simulink model "Coupled_GP_fit"  (R2018b)
settings: Solver=FixedStepAuto  StartTime=0.0  StopTime=t_end  FixedStep=ts  MinStep=1/1e5  RelTol=1e-3
values from neighbouring files (symbols this model uses):
  a0 = omega_n^3    (= 248050213.442)    [TwoLink_init.m]    (also in init.m = 31006276.6803)
  a1 = 3*omega_n^2    (= 1184352.52813)    [TwoLink_init.m]    (also in init.m = 296088.132033)
  a2 = 3*omega_n    (= 1884.95559215)    [TwoLink_init.m]    (also in init.m = 942.477796077)
  b1 = b(:,1)    [init.m]
  b2 = b(:,2)    [init.m]
  D = 50    [Train_SSGP.m]    (also in init.m = 21)
  g = 9.81    [init.m]
  h = 1    [init.m]
  I_limit = 2000    [TwoLink_init.m]
  L1 = 1    [init.m]
  L2 = 1    [init.m]
  m1 = 1    [init.m]
  m2 = 5    [init.m]
  mu_X = mean(xTrain')    [Train_SSGP.m]    (also in init.m = zeros(1,size(n,2)))
  mu_Y = mean(yTrain')    [Train_SSGP.m]    (also in init.m = zeros(1,size(Q,2)))
  N = size(xTrain,2)    [Train_SSGP.m]    (also in init.m = length(noiseSignal))
  r = 5e3    (= 5000)    [init.m]
  R1 = squeeze(R(1,:,:))    [init.m]
  R2 = squeeze(R(2,:,:))    [init.m]
  s = xTrain(:,i_s)'    [Train_SSGP.m]    (also in TwoLink_init.m = tf('s'))
  seed = randi(1e6)    [init.m]
  sf1 = sf(1)    [init.m]
  sf2 = sf(2)    [init.m]
  sig_X = std(xTrain')    [Train_SSGP.m]    (also in init.m = ones(1,size(n,2)))
  sig_Y = std(yTrain')    [Train_SSGP.m]    (also in init.m = ones(1,size(n,2)))
  SIGMA1 = squeeze(SIGMA(1,:,:))    [init.m]
  SIGMA2 = squeeze(SIGMA(2,:,:))    [init.m]
  sp_ts = 2.5    [init.m]
  t_learn = 0    [init.m]
  t_predict = 50    [init.m]
  tm = 2    [init.m]
  ts = 1/1000    (= 0.001)    [Train_SSGP.m]    (also in TwoLink_init.m; init.m)
  w1 = w(:,1)    [init.m]
  w2 = w(:,2)    [init.m]
  X = squeeze(xTraining(:,1,:))'    [init.m]    (also in plot_train_data.m = squeeze(input_vector.Data(:,:,ts_index)))
  Y = yTraining    [init.m]
undefined symbols (not defined in the file or in its folder): DiscIntNeverNeededParam, FF, noise, PID, Z
libraries: sm_lib x13, simulink x6, nesl_utility x5
(part 1 of 2)
settings Model: Creator=wout7  LastModifiedBy=wout7
settings DataIOCC: SaveFormat=StructureWithTime
settings OptimizationCC: BlockReduction=off  EfficientMapNaN2IntZero=off  SimCompilerOptimization=on
settings HardwareCC: TargetBitPerPointer=64  TargetBitPerSizeT=64  TargetBitPerPtrDiffT=64  TargetLongLongMode=on  TargetIntDivRoundTo=Zero  TargetEndianess=LittleEndian  TargetWordSize=64  TargetHWDeviceType=MATLAB Host  ProdEqTarget=off
settings SFSimCC: SimCustomSourceCode=solve_chol.c  MATLABDynamicMemAllocThreshold=98304
settings CodeAppCC: MaxIdLength=128
settings GRTTargetCC: TargetLangStandard=C89/C90 (ANSI)  CombineOutputUpdateFcns=off  GRTInterface=on

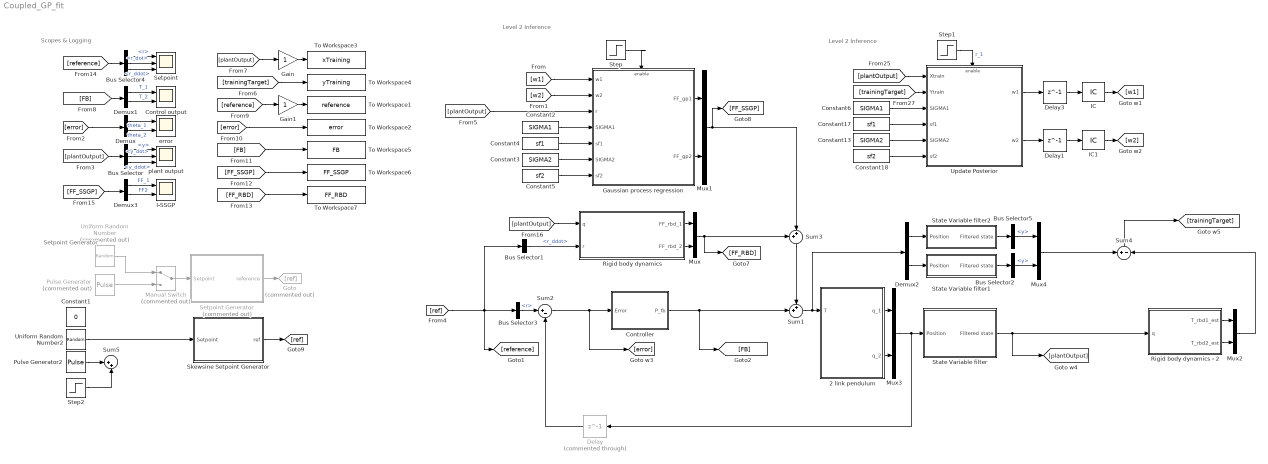
== system Coupled_GP_fit ==
  note: Level 2 Inference
  note: Scopes & Logging
  note: Level 2 Inference
  note: Setpoint Generator
  2 link pendulum : Subsystem
  Bus Selector : BusSelector  OutputSignals=y,y_dot,y_ddot
  Bus Selector1 : BusSelector  OutputSignals=r_ddot
  Bus Selector2 : BusSelector  OutputSignals=y
  Bus Selector3 : BusSelector  OutputSignals=r
  Bus Selector4 : BusSelector  OutputSignals=r,r_dot,r_ddot
  Bus Selector5 : BusSelector  OutputSignals=y
  Constant1 : Constant  Value=0  SampleTime=sp_ts
  Constant13 : Constant  Value=SIGMA2
  Constant17 : Constant  Value=sf1
  Constant18 : Constant  Value=sf2
  Constant2 : Constant  Value=SIGMA1
  Constant3 : Constant  Value=SIGMA2
  Constant4 : Constant  Value=sf1
  Constant5 : Constant  Value=sf2
  Constant6 : Constant  Value=SIGMA1
  Control output : Scope  NumInputPorts=2
  Controller : Subsystem
  Delay : Delay  Commented=through  DelayLength=1  InitialCondition=0
  Delay1 : Delay  DelayLength=1  InitialCondition=0
  Delay3 : Delay  DelayLength=1  InitialCondition=0
  Demux{,1..3} (4 alike) : Demux  Outputs=2
  Gain : Gain
  Gain1 : Gain
  Gaussian process regression : Subsystem
  Goto : Goto  Commented=on  GotoTag=ref
  I-SSGP : Scope  NumInputPorts=2
  IC : InitialCondition  Value=w1
  IC1 : InitialCondition  Value=w2
  Manual Switch : ManualSwitch  Commented=on
  Mux{,1..4} (5 alike) : Mux  Inputs=2
  Pulse Generator : DiscretePulseGenerator  Commented=on  PulseType=Time based  Amplitude=20*pi/180  Period=sp_ts  PulseWidth=50
  Pulse Generator2 : DiscretePulseGenerator  Amplitude=80*pi/180  Period=4  PulseWidth=2  SampleTime=sp_ts
  Rigid body dynamics : Subsystem
  Rigid body dynamics - 2 : Subsystem
  Setpoint : Scope  NumInputPorts=3
  Setpoint Generator : Subsystem  Commented=on
  Skewsine Setpoint Generator : Subsystem
  State Variable filter : Subsystem
  State Variable filter1 : Subsystem
  State Variable filter2 : Subsystem
  Step : Step  Time=t_predict  SampleTime=ts
  Step1 : Step  Time=t_learn  SampleTime=ts
  Step2 : Step  Time=sp_ts  After=-40*pi/180  SampleTime=sp_ts
  Sum1 : Sum  Inputs=++|
  Sum2 : Sum  Inputs=|+-
  Sum3 : Sum  Inputs=++|
  Sum4 : Sum  Inputs=+|-
  Sum5 : Sum  Inputs=|++
  To Workspace1 : ToWorkspace  VariableName=reference  SampleTime=-1
  To Workspace2 : ToWorkspace  VariableName=error  SampleTime=-1
  To Workspace3 : ToWorkspace  VariableName=xTraining  SampleTime=-1
  To Workspace4 : ToWorkspace  VariableName=yTraining  SampleTime=-1
  To Workspace5 : ToWorkspace  VariableName=FB  SampleTime=-1
  To Workspace6 : ToWorkspace  VariableName=FF_SSGP  SampleTime=-1
  To Workspace7 : ToWorkspace  VariableName=FF_RBD  SampleTime=-1
  Uniform Random Number : UniformRandomNumber  Commented=on  Minimum=-50*pi/180  Maximum=50*pi/180  Seed=seed  SampleTime=sp_ts
  Uniform Random Number2 : UniformRandomNumber  Minimum=-50*pi/180  Maximum=50*pi/180  Seed=seed  SampleTime=sp_ts
  Update Posterior : Subsystem
  error : Scope  NumInputPorts=2
  plant output : Scope  NumInputPorts=3
  wires:
  2 link pendulum/1(q_1) -> Mux3/1
  2 link pendulum/2(q_2) -> Mux3/2
  Sum1/1 -> Demux2/1, 2 link pendulum/1(T)
  Rigid body dynamics/1(FF_rbd_1) -> Mux/1
  Rigid body dynamics/2(FF_rbd_2) -> Mux/2
  Rigid body dynamics - 2/1(T_rbd1_est) -> Mux2/1
  Rigid body dynamics - 2/2(T_rbd2_est) -> Mux2/2
  Mux1/1 -> Sum3/2, [FF_SSGP]
  Sum4/1 -> [trainingTarget]
  Gaussian process regression/2(FF_gp2) -> Mux1/2
  Gaussian process regression/1(FF_gp1) -> Mux1/1
  Step/1 -> Gaussian process regression/Enable
  [w1] -> Gaussian process regression/1(w1)
  Update Posterior/1(w1) -> Delay3/1
  IC/1 -> [w1]
  IC1/1 -> [w2]
  [w2] -> Gaussian process regression/2(w2)
  Update Posterior/2(w2) -> Delay1/1
  Delay3/1 -> IC/1
  Delay1/1 -> IC1/1
  Mux2/1 -> Sum4/2
  Pulse Generator/1 -> Manual Switch/2
  Uniform Random Number/1 -> Manual Switch/1
  Controller/1(P_fb) -> Sum1/2, [FB]
  Mux/1 -> Sum3/1, [FF_RBD]
  [ref] -> Bus Selector1/1, [reference], Bus Selector3/1
  Sum3/1 -> Sum1/1
  Mux3/1 -> Delay/1, State Variable filter/1(Position)
  Bus Selector3/1 -> Sum2/1  "<r>"
  Bus Selector1/1 -> Rigid body dynamics/2(r)  "<r_ddot>"
  Setpoint Generator/1(reference) -> Goto/1
  Manual Switch/1 -> Setpoint Generator/1(Setpoint)
  Sum2/1 -> Controller/1(Error), [error]
  Delay/1 -> Sum2/2
  Step1/1 -> Update Posterior/Enable  "r_1"
  [plantOutput] -> Bus Selector/1
  Bus Selector/1 -> plant output/1  "<y>"
  Bus Selector/2 -> plant output/2  "<y_dot>"
  Bus Selector/3 -> plant output/3  "<y_ddot>"
  [error] -> Demux/1
  Demux/1 -> error/1  "theta_1"
  Demux/2 -> error/2  "theta_2"
  [trainingTarget] -> To Workspace4/1
  [plantOutput] -> Gain/1
  [reference] -> Gain1/1
  Demux1/1 -> Control output/1  "T_1"
  Demux1/2 -> Control output/2  "T_2"
  [FB] -> Demux1/1
  Gain/1 -> To Workspace3/1
  Gain1/1 -> To Workspace1/1
  [error] -> To Workspace2/1
  [FB] -> To Workspace5/1
  [FF_SSGP] -> To Workspace6/1
  [FF_RBD] -> To Workspace7/1
  [reference] -> Bus Selector4/1
  Bus Selector4/1 -> Setpoint/1  "<r>"
  Bus Selector4/2 -> Setpoint/2  "<r_dot>"
  Bus Selector4/3 -> Setpoint/3  "<r_ddot>"
  Skewsine Setpoint Generator/1(ref) -> [ref]
  Pulse Generator2/1 -> Sum5/1
  Step2/1 -> Sum5/2
  Uniform Random Number2/1 -> Skewsine Setpoint Generator/1(Setpoint)
  State Variable filter/1(Filtered state) -> Rigid body dynamics - 2/1(q), [plantOutput]
  Demux3/2 -> I-SSGP/2  "FF2"
  Demux3/1 -> I-SSGP/1  "FF_1"
  [FF_SSGP] -> Demux3/1
  Constant2/1 -> Gaussian process regression/4(SIGMA1)
  Constant4/1 -> Gaussian process regression/5(sf1)
  Constant6/1 -> Update Posterior/3(SIGMA1)
  Constant17/1 -> Update Posterior/4(sf1)
  Constant13/1 -> Update Posterior/5(SIGMA2)
  Constant18/1 -> Update Posterior/6(sf2)
  Constant3/1 -> Gaussian process regression/6(SIGMA2)
  Constant5/1 -> Gaussian process regression/7(sf2)
  [plantOutput] -> Update Posterior/1(Xtrain)
  [trainingTarget] -> Update Posterior/2(Ytrain)
  [plantOutput] -> Rigid body dynamics/1(q)
  State Variable filter1/1(Filtered state) -> Bus Selector2/1
  Mux4/1 -> Sum4/1
  Demux2/1 -> State Variable filter2/1(Position)
  Demux2/2 -> State Variable filter1/1(Position)
  Bus Selector5/1 -> Mux4/1  "<y>"
  State Variable filter2/1(Filtered state) -> Bus Selector5/1
  Bus Selector2/1 -> Mux4/2  "<y>"
  [plantOutput] -> Gaussian process regression/3(r)

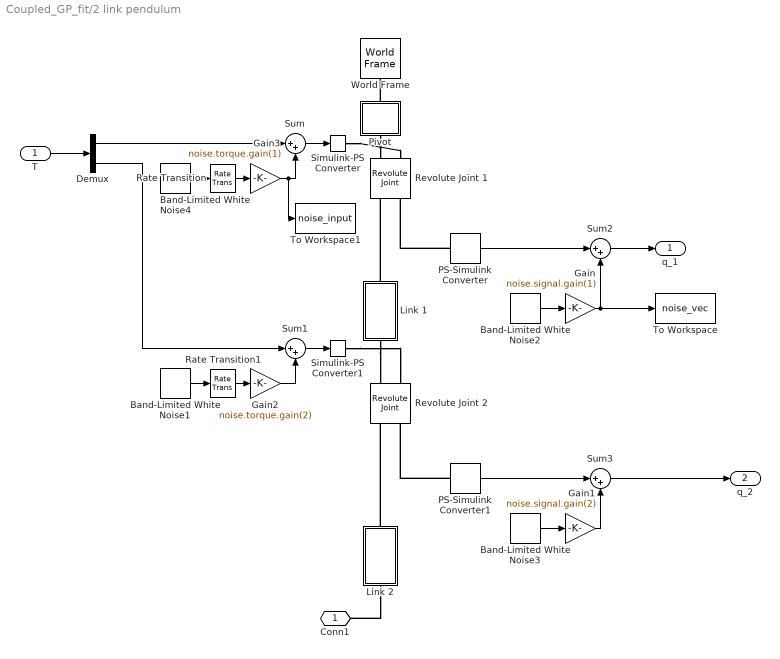
== system Coupled_GP_fit/2 link pendulum ==
  T : Inport
  Band-Limited White Noise1 : simulink/Sources/Band-Limited White Noise  Cov=noise.torque.power(2)  Ts=noise.sampleTime(1)  seed=[23341]
  Band-Limited White Noise2 : simulink/Sources/Band-Limited White Noise  Cov=noise.signal.power(1)  Ts=noise.sampleTime(2)  seed=[23341]
  Band-Limited White Noise3 : simulink/Sources/Band-Limited White Noise  Cov=noise.signal.power(2)  Ts=noise.sampleTime(2)  seed=[23341]
  Band-Limited White Noise4 : simulink/Sources/Band-Limited White Noise  Cov=noise.torque.power(1)  Ts=noise.sampleTime(1)  seed=[23341]
  Demux : Demux  Outputs=2
  Gain : Gain  Gain=noise.signal.gain(1)
  Gain1 : Gain  Gain=noise.signal.gain(2)
  Gain2 : Gain  Gain=noise.torque.gain(2)
  Gain3 : Gain  Gain=noise.torque.gain(1)
  Link 1 : Subsystem  Tag=CustomStyle
  Link 2 : Subsystem  Tag=CustomStyle
  PS-Simulink Converter : nesl_utility/PS-Simulink Converter  PhysicalDomain=network_engine_domain  SubClassName=ps_output  LeftPortType=input  RightPortType=output  PseudoPeriodic=off  Frequencies=[]  Unit=rad  AffineConversion=off
  PS-Simulink Converter1 : nesl_utility/PS-Simulink Converter  PhysicalDomain=network_engine_domain  SubClassName=ps_output  LeftPortType=input  RightPortType=output  PseudoPeriodic=off  Frequencies=[]  Unit=rad  AffineConversion=off
  Pivot : Subsystem  Tag=CustomStyle
  Rate Transition : RateTransition  OutPortSampleTime=ts
  Rate Transition1 : RateTransition  OutPortSampleTime=ts
  Revolute Joint 1 : sm_lib/Joints/Revolute Joint  SenseConstraintForce=off  SenseConstraintForceX=off  SenseConstraintForceY=off  SenseConstraintForceZ=off  SenseConstraintTorque=off  SenseConstraintTorqueX=off  SenseConstraintTorqueY=off  SenseConstraintTorqueZ=off  SenseTotalForce=off  SenseTotalForceX=off  SenseTotalForceY=off  SenseTotalForceZ=off  SenseTotalTorque=off  SenseTotalTorqueX=off  SenseTotalTorqueY=off  SenseTotalTorqueZ=off  CompositeWrenchDir=FollowerOnBase  CompositeWrenchFrame=BaseFrame  EquilibriumPosition=0  EquilibriumPositionUnits=rad  SpringStiffness=C_k1  SpringStiffnessUnits=N*m/rad  DampingCoefficient=C_d1  DampingCoefficientUnits=N*m/(rad/s)  TorqueActuationMode=InputTorque  MotionActuationMode=ComputedMotion  SensePosition=on  SenseVelocity=off  SenseAcceleration=off  SenseTorqueForce=off  PositionTargetSpecify=on  PositionTargetPriority=High  PositionTargetValue=theta1_0  PositionTargetValueUnits=deg  VelocityTargetSpecify=off  VelocityTargetPriority=High  VelocityTargetValue=0  VelocityTargetValueUnits=rad/s
  Revolute Joint 2 : sm_lib/Joints/Revolute Joint  SenseConstraintForce=off  SenseConstraintForceX=off  SenseConstraintForceY=off  SenseConstraintForceZ=off  SenseConstraintTorque=off  SenseConstraintTorqueX=off  SenseConstraintTorqueY=off  SenseConstraintTorqueZ=off  SenseTotalForce=off  SenseTotalForceX=off  SenseTotalForceY=off  SenseTotalForceZ=off  SenseTotalTorque=off  SenseTotalTorqueX=off  SenseTotalTorqueY=off  SenseTotalTorqueZ=off  CompositeWrenchDir=FollowerOnBase  CompositeWrenchFrame=BaseFrame  EquilibriumPosition=0  EquilibriumPositionUnits=rad  SpringStiffness=C_k1  SpringStiffnessUnits=N*m/rad  DampingCoefficient=C_d1  DampingCoefficientUnits=N*m/(rad/s)  TorqueActuationMode=InputTorque  MotionActuationMode=ComputedMotion  SensePosition=on  SenseVelocity=off  SenseAcceleration=off  SenseTorqueForce=off  PositionTargetSpecify=on  PositionTargetPriority=High  PositionTargetValue=theta2_0  PositionTargetValueUnits=deg  VelocityTargetSpecify=off  VelocityTargetPriority=High  VelocityTargetValue=0  VelocityTargetValueUnits=rad/s
  Simulink-PS Converter : nesl_utility/Simulink-PS Converter  PhysicalDomain=network_engine_domain  SubClassName=ps_input  LeftPortType=input  RightPortType=output  PseudoPeriodic=off  Frequencies=[]  NoiseDistribution=none  NoiseParameters=[]  Unit=1  AffineConversion=off  FilteringAndDerivatives=provide  SimscapeFilterOrder=1  InputFilterTimeConstant=0.001  UdotUserProvided=0
  Simulink-PS Converter1 : nesl_utility/Simulink-PS Converter  PhysicalDomain=network_engine_domain  SubClassName=ps_input  LeftPortType=input  RightPortType=output  PseudoPeriodic=off  Frequencies=[]  NoiseDistribution=none  NoiseParameters=[]  Unit=1  AffineConversion=off  FilteringAndDerivatives=provide  SimscapeFilterOrder=1  InputFilterTimeConstant=0.001  UdotUserProvided=0
  Sum{,1..3} (4 alike) : Sum  Inputs=|++
  To Workspace : ToWorkspace  VariableName=noise_vec  SaveFormat=Timeseries  SampleTime=-1
  To Workspace1 : ToWorkspace  VariableName=noise_input  SaveFormat=Timeseries  SampleTime=-1
  World Frame : sm_lib/Frames and Transforms/World Frame
  Conn1 : PMIOPort  Side=Left
  q_1 : Outport  SampleTime=ts
  q_2 : Outport  Port=2  SampleTime=ts
  wires:
  T/1 -> Demux/1
  Band-Limited White Noise1/1 -> Rate Transition1/1
  Demux/1 -> Sum/1
  Sum/1 -> Simulink-PS Converter/1
  Demux/2 -> Sum1/1
  Band-Limited White Noise2/1 -> Gain/1
  Sum2/1 -> q_1/1
  Band-Limited White Noise3/1 -> Gain1/1
  Sum3/1 -> q_2/1
  Gain/1 -> To Workspace/1, Sum2/2
  Gain1/1 -> Sum3/2
  Gain2/1 -> Sum1/2
  Gain3/1 -> Sum/2, To Workspace1/1
  Sum1/1 -> Simulink-PS Converter1/1
  Band-Limited White Noise4/1 -> Rate Transition/1
  Rate Transition/1 -> Gain3/1
  Rate Transition1/1 -> Gain2/1
  PS-Simulink Converter/1 -> Sum2/1
  PS-Simulink Converter1/1 -> Sum3/1
  connections:
  PS-Simulink Converter/LConn1 -- Revolute Joint 1/RConn2
  Link 2/RConn1 -- Revolute Joint 2/RConn1
  Pivot/LConn1 -- World Frame/RConn1
  Simulink-PS Converter/RConn1 -- Revolute Joint 1/LConn2
  Link 1/RConn1 -- Revolute Joint 1/RConn1
  Pivot/RConn1 -- Revolute Joint 1/LConn1
  PS-Simulink Converter1/LConn1 -- Revolute Joint 2/RConn2
  Link 1/LConn1 -- Revolute Joint 2/LConn1
  Link 2/LConn1 -- Conn1/RConn1
  Simulink-PS Converter1/RConn1 -- Revolute Joint 2/LConn2

== system Coupled_GP_fit/Controller ==
  Error : Inport
  Demux : Demux  Outputs=2
  Demux1 : Demux  Commented=on  Outputs=2
  Goto : Goto  Commented=on
  Mux : Mux  Inputs=2
  Mux1 : Mux  Commented=on  Inputs=2
  PID 1 : Subsystem  Commented=on
  PID 2 : Subsystem  Commented=on
  PID Controller : simulink/Continuous/PID Controller  Controller=PID  Form=Parallel  TimeDomain=Discrete-time  SampleTime=-1  IntegratorMethod=Forward Euler  FilterMethod=Forward Euler  ControllerParametersSource=internal  P=PID(1).kp*PID(1).sign*PID(1).sign  I=PID(1).ki*PID(1).sign  D=PID(1).kd*PID(1).sign  UseFilter=on  N=PID(1).N*PID(1).sign  TunerSelectOption=Transfer Function Based (PID Tuner App)  InitialConditionSource=internal  InitialConditionForIntegrator=0  InitialConditionForFilter=0  DifferentiatorICPrevScaledInput=0  ExternalReset=none  TrackingMode=off  Kt=1  LimitOutput=off  UpperSaturationLimit=inf  LowerSaturationLimit=-inf  LinearizeAsGain=on  AntiWindupMode=none  Kb=1  POutMin=[]  POutMax=[]  IOutMin=[]  IOutMax=[]  DOutMin=[]  DOutMax=[]  NOutMin=[]  NOutMax=[]  SumOutMin=[]  SumOutMax=[]  SaturationOutMin=[]  SaturationOutMax=[]  PParamMin=[]  PParamMax=[]  IParamMin=[]  IParamMax=[]  DParamMin=[]  DParamMax=[]  NParamMin=[]  NParamMax=[]  KbParamMin=[]  KbParamMax=[]  KtParamMin=[]  KtParamMax=[]  KbOutMin=[]  KbOutMax=[]  KtOutMin=[]  KtOutMax=[]  IntegratorOutMin=[]  IntegratorOutMax=[]  FilterOutMin=[]  FilterOutMax=[]  SumI1OutMin=[]  SumI1OutMax=[]  SumI2OutMin=[]  SumI2OutMax=[]  SumI3OutMin=[]  SumI3OutMax=[]  SumI4OutMin=[]  SumI4OutMax=[]  SumDOutMin=[]  SumDOutMax=[]  DifferentiatorOutMin=[]  DifferentiatorOutMax=[]  FilterDiffOutCoefMin=[]  FilterDiffOutCoefMax=[]  ReciprocalOutMin=[]  ReciprocalOutMax=[]  SumDenOutMin=[]  SumDenOutMax=[]  SumNumOutMin=[]  SumNumOutMax=[]  DivideOutMin=[]  DivideOutMax=[]  IntegratorContinuousStateAttributes=''  IntegratorStateMustResolveToSignalObject=off  IntegratorRTWStateStorageClass=Auto  FilterContinuousStateAttributes=''  FilterStateMustResolveToSignalObject=off  FilterRTWStateStorageClass=Auto  ParallelPVariant=InternalParameters  IdealPVariant=Disabled  IVariant=InternalParameters  DVariant=InternalParameters  IntegratorVariant=Discrete  SatVariant=Disabled  AWVariant=Passthrough  PCopyVariant=Disabled  TRVariant=Disabled  FdbkBlocksVariant=Forward  IdealPFdbkVariant=Disabled  SatFdbkVariant=Disabled  DerivativeFilterVariant=ForwardEulerFilter  NVariant=InternalParameters  NCopyVariant=Disabled  FilterICVariant=InternalICsFilter  IntegratorICVariant=InternalICs  ExternalResetVariant=Disabled  TRSumVariant=Passthrough  SumFdbkVariant=Disabled  SumVariant=Sum_PID
  PID Controller1 : simulink/Continuous/PID Controller  Controller=PID  Form=Parallel  TimeDomain=Discrete-time  SampleTime=-1  IntegratorMethod=Forward Euler  FilterMethod=Forward Euler  ControllerParametersSource=internal  P=PID(2).kp*PID(2).sign*PID(2).sign  I=PID(2).ki*PID(2).sign  D=PID(2).kd*PID(2).sign  UseFilter=on  N=PID(2).N*PID(2).sign  TunerSelectOption=Transfer Function Based (PID Tuner App)  InitialConditionSource=internal  InitialConditionForIntegrator=0  InitialConditionForFilter=0  DifferentiatorICPrevScaledInput=0  ExternalReset=none  TrackingMode=off  Kt=1  LimitOutput=off  UpperSaturationLimit=inf  LowerSaturationLimit=-inf  LinearizeAsGain=on  AntiWindupMode=none  Kb=1  POutMin=[]  POutMax=[]  IOutMin=[]  IOutMax=[]  DOutMin=[]  DOutMax=[]  NOutMin=[]  NOutMax=[]  SumOutMin=[]  SumOutMax=[]  SaturationOutMin=[]  SaturationOutMax=[]  PParamMin=[]  PParamMax=[]  IParamMin=[]  IParamMax=[]  DParamMin=[]  DParamMax=[]  NParamMin=[]  NParamMax=[]  KbParamMin=[]  KbParamMax=[]  KtParamMin=[]  KtParamMax=[]  KbOutMin=[]  KbOutMax=[]  KtOutMin=[]  KtOutMax=[]  IntegratorOutMin=[]  IntegratorOutMax=[]  FilterOutMin=[]  FilterOutMax=[]  SumI1OutMin=[]  SumI1OutMax=[]  SumI2OutMin=[]  SumI2OutMax=[]  SumI3OutMin=[]  SumI3OutMax=[]  SumI4OutMin=[]  SumI4OutMax=[]  SumDOutMin=[]  SumDOutMax=[]  DifferentiatorOutMin=[]  DifferentiatorOutMax=[]  FilterDiffOutCoefMin=[]  FilterDiffOutCoefMax=[]  ReciprocalOutMin=[]  ReciprocalOutMax=[]  SumDenOutMin=[]  SumDenOutMax=[]  SumNumOutMin=[]  SumNumOutMax=[]  DivideOutMin=[]  DivideOutMax=[]  IntegratorContinuousStateAttributes=''  IntegratorStateMustResolveToSignalObject=off  IntegratorRTWStateStorageClass=Auto  FilterContinuousStateAttributes=''  FilterStateMustResolveToSignalObject=off  FilterRTWStateStorageClass=Auto  ParallelPVariant=InternalParameters  IdealPVariant=Disabled  IVariant=InternalParameters  DVariant=InternalParameters  IntegratorVariant=Discrete  SatVariant=Disabled  AWVariant=Passthrough  PCopyVariant=Disabled  TRVariant=Disabled  FdbkBlocksVariant=Forward  IdealPFdbkVariant=Disabled  SatFdbkVariant=Disabled  DerivativeFilterVariant=ForwardEulerFilter  NVariant=InternalParameters  NCopyVariant=Disabled  FilterICVariant=InternalICsFilter  IntegratorICVariant=InternalICs  ExternalResetVariant=Disabled  TRSumVariant=Passthrough  SumFdbkVariant=Disabled  SumVariant=Sum_PID
  P_fb : Outport
  wires:
  Demux/2 -> PID Controller1/1
  Demux/1 -> PID Controller/1
  Error/1 -> Demux1/1, Demux/1
  PID Controller1/1 -> Mux/2  "T_fb2"
  PID Controller/1 -> Mux/1  "T_fb1"
  Demux1/1 -> PID 1/1(In1)
  Demux1/2 -> PID 2/1(In1)
  PID 1/1(Out1) -> Mux1/1
  PID 2/1(Out1) -> Mux1/2
  Mux1/1 -> Goto/1
  [A] -> P_fb/1
  Mux/1 -> [A]

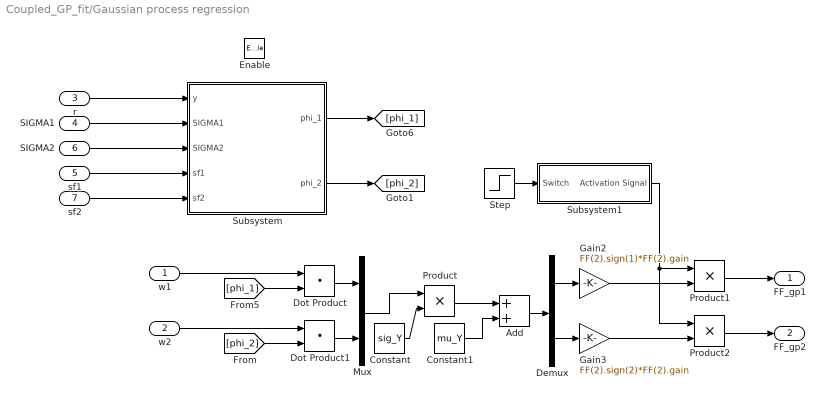
== system Coupled_GP_fit/Gaussian process regression ==
  w1 : Inport
  w2 : Inport  Port=2
  r : Inport  Port=3
  SIGMA1 : Inport  Port=4
  sf1 : Inport  Port=5
  SIGMA2 : Inport  Port=6
  sf2 : Inport  Port=7
  Enable : EnablePort
  Add : Sum
  Constant : Constant  Value=sig_Y  VectorParams1D=off  SampleTime=ts
  Constant1 : Constant  Value=mu_Y  VectorParams1D=off  SampleTime=ts
  Demux : Demux  Outputs=2
  Dot Product : DotProduct  OutDataTypeStr=Inherit: Inherit via internal rule
  Dot Product1 : DotProduct  OutDataTypeStr=Inherit: Inherit via internal rule
  Gain2 : Gain  Gain=FF(2).sign(1)*FF(2).gain
  Gain3 : Gain  Gain=FF(2).sign(2)*FF(2).gain
  Mux : Mux  Inputs=2
  Product : Product
  Product1 : Product
  Product2 : Product
  Step : Step  Time=t_predict  SampleTime=ts
  Subsystem : Subsystem
  Subsystem1 : Subsystem
  FF_gp1 : Outport  SampleTime=ts
  FF_gp2 : Outport  Port=2  SampleTime=ts
  wires:
  w1/1 -> Dot Product/1
  w2/1 -> Dot Product1/1
  [phi_2] -> Dot Product1/2
  [phi_1] -> Dot Product/2
  SIGMA2/1 -> Subsystem/3(SIGMA2)
  Subsystem/1(phi_1) -> [phi_1]
  Subsystem/2(phi_2) -> [phi_2]
  Dot Product1/1 -> Mux/2
  Dot Product/1 -> Mux/1
  Constant/1 -> Product/2
  Mux/1 -> Product/1
  Demux/1 -> Gain2/1
  Demux/2 -> Gain3/1
  Add/1 -> Demux/1
  Product/1 -> Add/1
  Constant1/1 -> Add/2
  r/1 -> Subsystem/1(y)
  Gain2/1 -> Product1/2
  Gain3/1 -> Product2/2
  Subsystem1/1(Activation Signal) -> Product2/1, Product1/1
  Product1/1 -> FF_gp1/1
  Product2/1 -> FF_gp2/1
  SIGMA1/1 -> Subsystem/2(SIGMA1)
  sf1/1 -> Subsystem/4(sf1)
  sf2/1 -> Subsystem/5(sf2)
  Step/1 -> Subsystem1/1(Switch)

== system Coupled_GP_fit/Rigid body dynamics ==
  q : Inport
  r : Inport  Port=2
  Bus Selector : BusSelector  OutputSignals=y
  Bus Selector1 : BusSelector  OutputSignals=y_dot
  Bus Selector2 : BusSelector  OutputSignals=y_ddot
  MATLAB Function : MATLAB Function  TreatAsAtomicUnit=on
  Sign - 1 : Gain  Gain=FF(1).sign*FF(1).gain
  Sign - 2 : Gain  Gain=FF(1).sign*FF(1).gain
  FF_rbd_1 : Outport
  FF_rbd_2 : Outport  Port=2
  wires:
  MATLAB Function/2(FF_rbd2) -> Sign - 2/1
  MATLAB Function/1(FF_rgd1) -> Sign - 1/1
  Sign - 1/1 -> FF_rbd_1/1
  Sign - 2/1 -> FF_rbd_2/1
  r/1 -> MATLAB Function/5(q_r_ddot)
  Bus Selector/1 -> MATLAB Function/1(q)  "<y>"
  Bus Selector1/1 -> MATLAB Function/4(q_r_dot), MATLAB Function/2(q_dot)  "<y_dot>"
  Bus Selector2/1 -> MATLAB Function/3(q_ddot)  "<y_ddot>"
  q/1 -> Bus Selector2/1, Bus Selector1/1, Bus Selector/1

== system Coupled_GP_fit/Rigid body dynamics - 2 ==
  q : Inport
  Bus Selector : BusSelector  OutputSignals=y
  Bus Selector1 : BusSelector  OutputSignals=y_dot
  Bus Selector2 : BusSelector  OutputSignals=y_ddot
  MATLAB Function : MATLAB Function  TreatAsAtomicUnit=on
  Sign - 1 : Gain  Gain=FF(1).sign(1)*FF(1).gain
  Sign - 2 : Gain  Gain=FF(2).sign(2)*FF(1).gain
  T_rbd1_est : Outport
  T_rbd2_est : Outport  Port=2
  wires:
  MATLAB Function/2(T_ff2) -> Sign - 2/1
  MATLAB Function/1(T_ff1) -> Sign - 1/1
  Sign - 1/1 -> T_rbd1_est/1
  Sign - 2/1 -> T_rbd2_est/1
  q/1 -> Bus Selector2/1, Bus Selector1/1, Bus Selector/1
  Bus Selector/1 -> MATLAB Function/1(q)  "<y>"
  Bus Selector1/1 -> MATLAB Function/4(q_r_dot), MATLAB Function/2(q_dot)  "<y_dot>"
  Bus Selector2/1 -> MATLAB Function/5(q_r_ddot), MATLAB Function/3(q_ddot)  "<y_ddot>"

== system Coupled_GP_fit/Setpoint Generator ==
  Setpoint : Inport
  Bus Creator : BusCreator  Inputs=3
  Bus Creator1 : BusCreator  Inputs=2
  Bus Creator2 : BusCreator  Inputs=2
  Bus Creator3 : BusCreator  Inputs=2
  Gain1 : Gain  Gain=-1
  TDfhan : Subsystem
  TDfhan1 : Subsystem
  reference : Outport
  wires:
  TDfhan1/1(V1) -> Bus Creator1/2  "x2"
  Setpoint/1 -> TDfhan/1(V), Gain1/1
  TDfhan1/2(V2) -> Bus Creator2/2  "v2"
  TDfhan/3(V3) -> Bus Creator3/1  "a1"
  Bus Creator/1 -> reference/1
  Gain1/1 -> TDfhan1/1(V)
  TDfhan1/3(V3) -> Bus Creator3/2  "a2"
  TDfhan/2(V2) -> Bus Creator2/1  "v1"
  TDfhan/1(V1) -> Bus Creator1/1  "x1"
  Bus Creator1/1 -> Bus Creator/1  "r"
  Bus Creator2/1 -> Bus Creator/2  "r_dot"
  Bus Creator3/1 -> Bus Creator/3  "r_ddot"

== system Coupled_GP_fit/Skewsine Setpoint Generator ==
  Setpoint : Inport
  Bus Creator : BusCreator  Inputs=3
  Bus Creator1 : BusCreator  Inputs=2
  Bus Creator2 : BusCreator  Inputs=2
  Bus Creator3 : BusCreator  Inputs=2
  Gain2 : Gain  Gain=-1
  Subsystem : Subsystem
  Subsystem1 : Subsystem
  ref : Outport
  wires:
  Subsystem/3(r_ddot) -> Bus Creator3/1  "a1"
  Subsystem1/3(r_ddot) -> Bus Creator3/2  "a2"
  Subsystem/1(r) -> Bus Creator1/1  "x1"
  Subsystem/2(r_dot) -> Bus Creator2/1  "v1"
  Subsystem1/1(r) -> Bus Creator1/2  "x2"
  Bus Creator/1 -> ref/1
  Subsystem1/2(r_dot) -> Bus Creator2/2  "v2"
  Setpoint/1 -> Subsystem/1(setpoint), Gain2/1
  Gain2/1 -> Subsystem1/1(setpoint)
  Bus Creator2/1 -> Bus Creator/2  "r_dot"
  Bus Creator3/1 -> Bus Creator/3  "r_ddot"
  Bus Creator1/1 -> Bus Creator/1  "r"

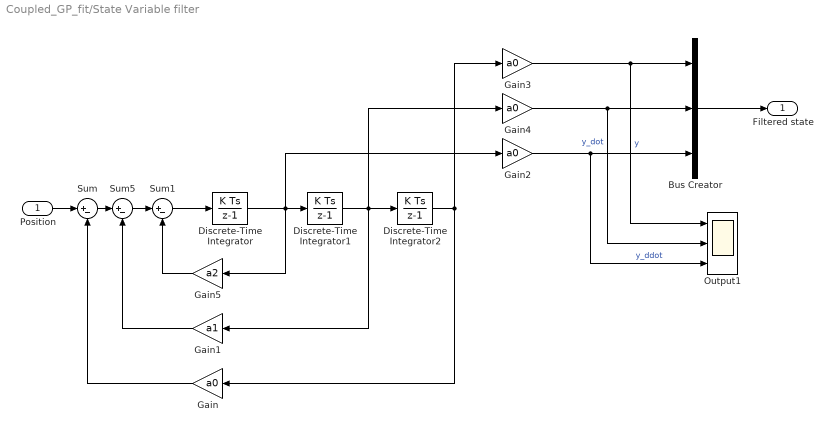
== system Coupled_GP_fit/State Variable filter ==
  Position : Inport
  Bus Creator : BusCreator  Inputs=3
  Discrete-Time Integrator : DiscreteIntegrator  SampleTime=ts  ICPrevOutput=DiscIntNeverNeededParam  ICPrevScaledInput=DiscIntNeverNeededParam
  Discrete-Time Integrator1 : DiscreteIntegrator  SampleTime=ts  ICPrevOutput=DiscIntNeverNeededParam  ICPrevScaledInput=DiscIntNeverNeededParam
  Discrete-Time Integrator2 : DiscreteIntegrator  SampleTime=ts  ICPrevOutput=DiscIntNeverNeededParam  ICPrevScaledInput=DiscIntNeverNeededParam
  Gain{,2..4} (4 alike) : Gain  Gain=a0
  Gain1 : Gain  Gain=a1
  Gain5 : Gain  Gain=a2
  Output1 : Scope  NumInputPorts=3
  Sum : Sum  Inputs=|+-
  Sum1 : Sum  Inputs=|+-
  Sum5 : Sum  Inputs=|+-
  Filtered state : Outport  SampleTime=ts
  wires:
  Bus Creator/1 -> Filtered state/1
  Sum1/1 -> Discrete-Time Integrator/1
  Position/1 -> Sum/1
  Sum/1 -> Sum5/1
  Gain/1 -> Sum/2
  Gain1/1 -> Sum5/2
  Gain3/1 -> Output1/1, Bus Creator/1  "y"
  Gain2/1 -> Output1/3, Bus Creator/3  "y_ddot"
  Gain4/1 -> Output1/2, Bus Creator/2  "y_dot"
  Gain5/1 -> Sum1/2
  Sum5/1 -> Sum1/1
  Discrete-Time Integrator/1 -> Discrete-Time Integrator1/1, Gain2/1, Gain5/1
  Discrete-Time Integrator1/1 -> Discrete-Time Integrator2/1, Gain4/1, Gain1/1
  Discrete-Time Integrator2/1 -> Gain3/1, Gain/1

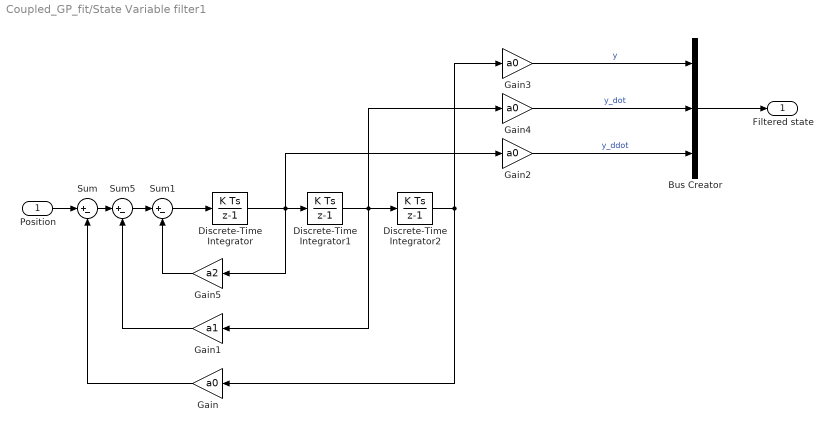
== system Coupled_GP_fit/State Variable filter1 ==
  Position : Inport
  Bus Creator : BusCreator  Inputs=3
  Discrete-Time Integrator : DiscreteIntegrator  SampleTime=ts  ICPrevOutput=DiscIntNeverNeededParam  ICPrevScaledInput=DiscIntNeverNeededParam
  Discrete-Time Integrator1 : DiscreteIntegrator  SampleTime=ts  ICPrevOutput=DiscIntNeverNeededParam  ICPrevScaledInput=DiscIntNeverNeededParam
  Discrete-Time Integrator2 : DiscreteIntegrator  SampleTime=ts  ICPrevOutput=DiscIntNeverNeededParam  ICPrevScaledInput=DiscIntNeverNeededParam
  Gain{,2..4} (4 alike) : Gain  Gain=a0
  Gain1 : Gain  Gain=a1
  Gain5 : Gain  Gain=a2
  Sum : Sum  Inputs=|+-
  Sum1 : Sum  Inputs=|+-
  Sum5 : Sum  Inputs=|+-
  Filtered state : Outport  SampleTime=ts
  wires:
  Bus Creator/1 -> Filtered state/1
  Sum1/1 -> Discrete-Time Integrator/1
  Position/1 -> Sum/1
  Sum/1 -> Sum5/1
  Gain/1 -> Sum/2
  Gain1/1 -> Sum5/2
  Gain3/1 -> Bus Creator/1  "y"
  Gain2/1 -> Bus Creator/3  "y_ddot"
  Gain4/1 -> Bus Creator/2  "y_dot"
  Gain5/1 -> Sum1/2
  Sum5/1 -> Sum1/1
  Discrete-Time Integrator/1 -> Discrete-Time Integrator1/1, Gain2/1, Gain5/1
  Discrete-Time Integrator1/1 -> Discrete-Time Integrator2/1, Gain4/1, Gain1/1
  Discrete-Time Integrator2/1 -> Gain3/1, Gain/1

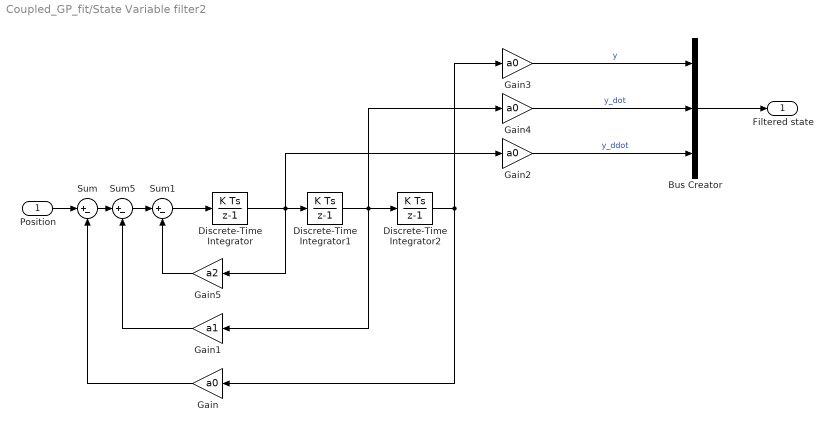
== system Coupled_GP_fit/State Variable filter2 ==
  Position : Inport
  Bus Creator : BusCreator  Inputs=3
  Discrete-Time Integrator : DiscreteIntegrator  SampleTime=ts  ICPrevOutput=DiscIntNeverNeededParam  ICPrevScaledInput=DiscIntNeverNeededParam
  Discrete-Time Integrator1 : DiscreteIntegrator  SampleTime=ts  ICPrevOutput=DiscIntNeverNeededParam  ICPrevScaledInput=DiscIntNeverNeededParam
  Discrete-Time Integrator2 : DiscreteIntegrator  SampleTime=ts  ICPrevOutput=DiscIntNeverNeededParam  ICPrevScaledInput=DiscIntNeverNeededParam
  Gain{,2..4} (4 alike) : Gain  Gain=a0
  Gain1 : Gain  Gain=a1
  Gain5 : Gain  Gain=a2
  Sum : Sum  Inputs=|+-
  Sum1 : Sum  Inputs=|+-
  Sum5 : Sum  Inputs=|+-
  Filtered state : Outport  SampleTime=ts
  wires:
  Bus Creator/1 -> Filtered state/1
  Sum1/1 -> Discrete-Time Integrator/1
  Position/1 -> Sum/1
  Sum/1 -> Sum5/1
  Gain/1 -> Sum/2
  Gain1/1 -> Sum5/2
  Gain3/1 -> Bus Creator/1  "y"
  Gain2/1 -> Bus Creator/3  "y_ddot"
  Gain4/1 -> Bus Creator/2  "y_dot"
  Gain5/1 -> Sum1/2
  Sum5/1 -> Sum1/1
  Discrete-Time Integrator/1 -> Discrete-Time Integrator1/1, Gain2/1, Gain5/1
  Discrete-Time Integrator1/1 -> Discrete-Time Integrator2/1, Gain4/1, Gain1/1
  Discrete-Time Integrator2/1 -> Gain3/1, Gain/1

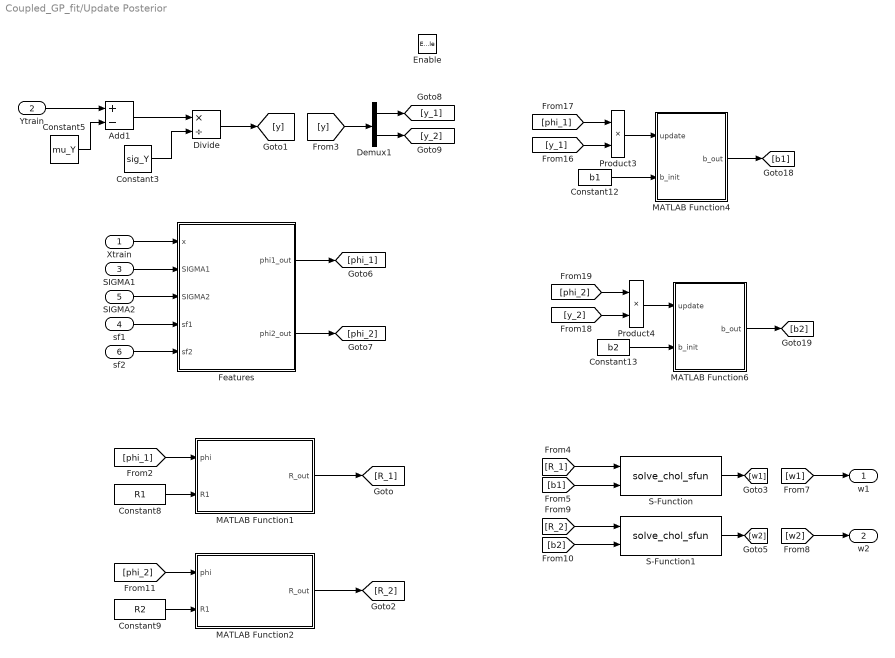
== system Coupled_GP_fit/Update Posterior ==
  Xtrain : Inport  SampleTime=ts
  Ytrain : Inport  Port=2  SampleTime=ts
  SIGMA1 : Inport  Port=3  SampleTime=ts
  sf1 : Inport  Port=4  SampleTime=ts
  SIGMA2 : Inport  Port=5  SampleTime=ts
  sf2 : Inport  Port=6  SampleTime=ts
  Enable : EnablePort
  Add1 : Sum  Inputs=+-
  Constant12 : Constant  Value=b1  VectorParams1D=off  SampleTime=ts
  Constant13 : Constant  Value=b2  VectorParams1D=off  SampleTime=ts
  Constant3 : Constant  Value=sig_Y  VectorParams1D=off  SampleTime=ts
  Constant5 : Constant  Value=mu_Y  VectorParams1D=off  SampleTime=ts
  Constant8 : Constant  Value=R1  VectorParams1D=off  SampleTime=ts
  Constant9 : Constant  Value=R2  VectorParams1D=off  SampleTime=ts
  Demux1 : Demux  Outputs=2
  Divide : Product  Inputs=*/
  Features : Subsystem
  MATLAB Function1 : MATLAB Function  TreatAsAtomicUnit=on
  MATLAB Function2 : MATLAB Function  TreatAsAtomicUnit=on
  MATLAB Function4 : MATLAB Function  TreatAsAtomicUnit=on
  MATLAB Function6 : MATLAB Function  TreatAsAtomicUnit=on
  Product3 : Product
  Product4 : Product
  S-Function : S-Function  FunctionName=solve_chol_sfun  Parameters=2*D  SFunctionDeploymentMode=off  EnableBusSupport=off
  S-Function1 : S-Function  FunctionName=solve_chol_sfun  Parameters=2*D  SFunctionDeploymentMode=off  EnableBusSupport=off
  w1 : Outport
  w2 : Outport  Port=2
  wires:
  Demux1/2 -> [y_2]
  Demux1/1 -> [y_1]
  [y] -> Demux1/1
  [phi_1] -> MATLAB Function1/1(phi)
  Xtrain/1 -> Features/1(x)
  Features/1(phi1_out) -> [phi_1]
  Features/2(phi2_out) -> [phi_2]
  MATLAB Function1/1(R_out) -> [R_1]
  SIGMA2/1 -> Features/3(SIGMA2)
  Ytrain/1 -> Add1/1
  Constant3/1 -> Divide/2
  Constant5/1 -> Add1/2
  Divide/1 -> [y]
  Add1/1 -> Divide/1
  [w1] -> w1/1
  [w2] -> w2/1
  Constant8/1 -> MATLAB Function1/2(R1)
  Constant9/1 -> MATLAB Function2/2(R1)
  [phi_2] -> MATLAB Function2/1(phi)
  MATLAB Function2/1(R_out) -> [R_2]
  [y_1] -> Product3/2
  [phi_1] -> Product3/1
  Product3/1 -> MATLAB Function4/1(update)
  Constant12/1 -> MATLAB Function4/2(b_init)
  MATLAB Function4/1(b_out) -> [b1]
  MATLAB Function6/1(b_out) -> [b2]
  Product4/1 -> MATLAB Function6/1(update)
  Constant13/1 -> MATLAB Function6/2(b_init)
  [phi_2] -> Product4/1
  [y_2] -> Product4/2
  SIGMA1/1 -> Features/2(SIGMA1)
  sf1/1 -> Features/4(sf1)
  sf2/1 -> Features/5(sf2)
  [R_1] -> S-Function/1
  [b1] -> S-Function/2
  S-Function/1 -> [w1]
  [b2] -> S-Function1/2
  S-Function1/1 -> [w2]
  [R_2] -> S-Function1/1

== system Coupled_GP_fit/2 link pendulum/Link 1 ==
  Bob : sm_lib/Body Elements/Solid  InertiaType=PointMass  Mass=0  MassUnits=kg  CenterOfMass=[0 0 0]  CenterOfMassUnits=m  MomentsOfInertia=[1 1 1]*1e-3  MomentsOfInertiaUnits=kg*m^2  ProductsOfInertia=[0 0 0]  ProductsOfInertiaUnits=kg*m^2  BasedOnType=Density  Density=1000  DensityUnits=kg/(m^3)  DoExposeReferenceFrame=on  SerializedFrames=<Frames/>  GraphicType=FromGeometry  MarkerShape=Sphere  MarkerSize=10  MarkerSizeUnits=m  GraphicVisPropType=SimpleVisualProperties  GraphicDiffuseColor=[1.0 0.2 0.0]  GraphicSpecularColor=[0.5 0.5 0.5 1.0]  GraphicAmbientColor=[0.15 0.15 0.15 1.0]  GraphicEmissiveColor=[0.0 0.0 0.0 1.0]  GraphicShininess=75  GraphicOpacity=1.0  GeometryShape=Sphere  RectangleSize=[1 1]  RectangleSizeUnits=m  BrickDimensions=[1 0.1 0.1]  BrickDimensionUnits=m  CylinderRadius=0.1  CylinderRadiusUnits=m  CylinderLength=1  CylinderLengthUnits=m  SphereRadius=0.1  SphereRadiusUnits=m  EllipsoidRadii=[1 1 1]  EllipsoidRadiiUnits=m  ExtrusionCrossSection=[1 1; -1 1; -1 -1; 1 -1]  ExtrusionCrossSectionUnits=m  ExtrusionLength=1  ExtrusionLengthUnits=m  PolygonNumSides=3  PolygonOuterRadius=1  PolygonOuterRadiusUnits=m  ExtGeomFileType=STL  ExtGeomFileUnits=m  RevolutionCrossSection=[1 1; 1 -1; 2 -1; 2 1]  RevolutionCrossSectionUnits=m  RevolutionExtent=Full  RevolutionAngle=180  RevolutionAngleUnits=deg
  String : sm_lib/Body Elements/Solid  InertiaType=CalculateFromGeometry  Mass=m1  MassUnits=kg  CenterOfMass=[0 0 0]  CenterOfMassUnits=m  MomentsOfInertia=[1 1 1]*1e-3  MomentsOfInertiaUnits=kg*m^2  ProductsOfInertia=[0 0 0]  ProductsOfInertiaUnits=kg*m^2  BasedOnType=Mass  Density=m1  DensityUnits=kg/(m^3)  DoExposeReferenceFrame=on  SerializedFrames=<Frames/>  GraphicType=FromGeometry  MarkerShape=Sphere  MarkerSize=10  MarkerSizeUnits=m  GraphicVisPropType=SimpleVisualProperties  GraphicDiffuseColor=[1.0 0.2 0.0]  GraphicSpecularColor=[0.5 0.5 0.5 1.0]  GraphicAmbientColor=[0.15 0.15 0.15 1.0]  GraphicEmissiveColor=[0.0 0.0 0.0 1.0]  GraphicShininess=75  GraphicOpacity=1.0  GeometryShape=Brick  RectangleSize=[1 1]  RectangleSizeUnits=m  BrickDimensions=[0.01 L1 0.01]  BrickDimensionUnits=m  CylinderRadius=0.1  CylinderRadiusUnits=m  CylinderLength=1  CylinderLengthUnits=m  SphereRadius=0.1  SphereRadiusUnits=m  EllipsoidRadii=[1 1 1]  EllipsoidRadiiUnits=m  ExtrusionCrossSection=[1 1; -1 1; -1 -1; 1 -1]  ExtrusionCrossSectionUnits=m  ExtrusionLength=1  ExtrusionLengthUnits=m  PolygonNumSides=3  PolygonOuterRadius=1  PolygonOuterRadiusUnits=m  ExtGeomFileType=STL  ExtGeomFileUnits=m  RevolutionCrossSection=[1 1; 1 -1; 2 -1; 2 1]  RevolutionCrossSectionUnits=m  RevolutionExtent=Full  RevolutionAngle=180  RevolutionAngleUnits=deg
  "Transform Bob " : sm_lib/Frames and Transforms/Rigid Transform  TranslationMethod=StandardAxis  TranslationStandardOffset=L1  TranslationLengthUnit=m  TranslationStandardAxis=-Y  TranslationCartesianOffset=[0 0 0]  TranslationROffset=0  TranslationROffsetUnits=m  TranslationZOffset=0  TranslationZOffsetUnits=m  TranslationThetaOffset=0  TranslationThetaOffsetUnits=deg  RotationMethod=None  RotationAngleUnits=deg  RotationStandardAxis=+Z  RotationAngle=0  RotationArbitraryAxis=[0 0 1]  FollAlignAxisA=+X  BaseAlignAxisA=+Y  FollAlignAxisB=+Y  BaseAlignAxisB=+Z  RotationSequenceAxes=FollowerAxes  RotationSequence=XYX  RotationSequenceAngles=[0 0 0]  RotationSequenceAnglesUnits=deg  RotationMatrix=[1 0 0; 0 1 0; 0 0 1]
  Transform String Midpoint : sm_lib/Frames and Transforms/Rigid Transform  TranslationMethod=StandardAxis  TranslationStandardOffset=L1/2  TranslationLengthUnit=m  TranslationStandardAxis=-Y  TranslationCartesianOffset=[0 0 0]  TranslationROffset=0  TranslationROffsetUnits=m  TranslationZOffset=0  TranslationZOffsetUnits=m  TranslationThetaOffset=0  TranslationThetaOffsetUnits=deg  RotationMethod=None  RotationAngleUnits=deg  RotationStandardAxis=+Z  RotationAngle=0  RotationArbitraryAxis=[0 0 1]  FollAlignAxisA=+X  BaseAlignAxisA=+Y  FollAlignAxisB=+Y  BaseAlignAxisB=+Z  RotationSequenceAxes=FollowerAxes  RotationSequence=XYX  RotationSequenceAngles=[0 0 0]  RotationSequenceAnglesUnits=deg  RotationMatrix=[1 0 0; 0 1 0; 0 0 1]
  B : PMIOPort  Side=Right
  F : PMIOPort  Port=2  Side=Left
  connections:
  "Transform Bob "/LConn1 -- Transform String Midpoint/LConn1 -- B/RConn1
  Bob/RConn1 -- F/RConn1 -- "Transform Bob "/RConn1
  Transform String Midpoint/RConn1 -- String/RConn1

== system Coupled_GP_fit/2 link pendulum/Link 2 ==
  Bob : sm_lib/Body Elements/Solid  InertiaType=PointMass  Mass=0  MassUnits=kg  CenterOfMass=[0 0 0]  CenterOfMassUnits=m  MomentsOfInertia=[1 1 1]*1e-3  MomentsOfInertiaUnits=kg*m^2  ProductsOfInertia=[0 0 0]  ProductsOfInertiaUnits=kg*m^2  BasedOnType=Density  Density=1000  DensityUnits=kg/(m^3)  DoExposeReferenceFrame=on  SerializedFrames=<Frames/>  GraphicType=FromGeometry  MarkerShape=Sphere  MarkerSize=10  MarkerSizeUnits=m  GraphicVisPropType=SimpleVisualProperties  GraphicDiffuseColor=[1.0 0.2 0.0]  GraphicSpecularColor=[0.5 0.5 0.5 1.0]  GraphicAmbientColor=[0.15 0.15 0.15 1.0]  GraphicEmissiveColor=[0.0 0.0 0.0 1.0]  GraphicShininess=75  GraphicOpacity=1.0  GeometryShape=Sphere  RectangleSize=[1 1]  RectangleSizeUnits=m  BrickDimensions=[1 0.1 0.1]  BrickDimensionUnits=m  CylinderRadius=0.1  CylinderRadiusUnits=m  CylinderLength=1  CylinderLengthUnits=m  SphereRadius=0.1  SphereRadiusUnits=m  EllipsoidRadii=[1 1 1]  EllipsoidRadiiUnits=m  ExtrusionCrossSection=[1 1; -1 1; -1 -1; 1 -1]  ExtrusionCrossSectionUnits=m  ExtrusionLength=1  ExtrusionLengthUnits=m  PolygonNumSides=3  PolygonOuterRadius=1  PolygonOuterRadiusUnits=m  ExtGeomFileType=STL  ExtGeomFileUnits=m  RevolutionCrossSection=[1 1; 1 -1; 2 -1; 2 1]  RevolutionCrossSectionUnits=m  RevolutionExtent=Full  RevolutionAngle=180  RevolutionAngleUnits=deg
  String : sm_lib/Body Elements/Solid  InertiaType=CalculateFromGeometry  Mass=m2  MassUnits=kg  CenterOfMass=[0 0 0]  CenterOfMassUnits=m  MomentsOfInertia=[1 1 1]*1e-3  MomentsOfInertiaUnits=kg*m^2  ProductsOfInertia=[0 0 0]  ProductsOfInertiaUnits=kg*m^2  BasedOnType=Mass  Density=0  DensityUnits=kg/(m^3)  DoExposeReferenceFrame=on  SerializedFrames=<Frames/>  GraphicType=FromGeometry  MarkerShape=Sphere  MarkerSize=10  MarkerSizeUnits=m  GraphicVisPropType=SimpleVisualProperties  GraphicDiffuseColor=[1.0 0.2 0.0]  GraphicSpecularColor=[0.5 0.5 0.5 1.0]  GraphicAmbientColor=[0.15 0.15 0.15 1.0]  GraphicEmissiveColor=[0.0 0.0 0.0 1.0]  GraphicShininess=75  GraphicOpacity=1.0  GeometryShape=Brick  RectangleSize=[1 1]  RectangleSizeUnits=m  BrickDimensions=[0.01 L2 0.01]  BrickDimensionUnits=m  CylinderRadius=0.1  CylinderRadiusUnits=m  CylinderLength=1  CylinderLengthUnits=m  SphereRadius=0.1  SphereRadiusUnits=m  EllipsoidRadii=[1 1 1]  EllipsoidRadiiUnits=m  ExtrusionCrossSection=[1 1; -1 1; -1 -1; 1 -1]  ExtrusionCrossSectionUnits=m  ExtrusionLength=1  ExtrusionLengthUnits=m  PolygonNumSides=3  PolygonOuterRadius=1  PolygonOuterRadiusUnits=m  ExtGeomFileType=STL  ExtGeomFileUnits=m  RevolutionCrossSection=[1 1; 1 -1; 2 -1; 2 1]  RevolutionCrossSectionUnits=m  RevolutionExtent=Full  RevolutionAngle=180  RevolutionAngleUnits=deg
  "Transform Bob " : sm_lib/Frames and Transforms/Rigid Transform  TranslationMethod=StandardAxis  TranslationStandardOffset=L2  TranslationLengthUnit=m  TranslationStandardAxis=-Y  TranslationCartesianOffset=[0 0 0]  TranslationROffset=0  TranslationROffsetUnits=m  TranslationZOffset=0  TranslationZOffsetUnits=m  TranslationThetaOffset=0  TranslationThetaOffsetUnits=deg  RotationMethod=None  RotationAngleUnits=deg  RotationStandardAxis=+Z  RotationAngle=0  RotationArbitraryAxis=[0 0 1]  FollAlignAxisA=+X  BaseAlignAxisA=+Y  FollAlignAxisB=+Y  BaseAlignAxisB=+Z  RotationSequenceAxes=FollowerAxes  RotationSequence=XYX  RotationSequenceAngles=[0 0 0]  RotationSequenceAnglesUnits=deg  RotationMatrix=[1 0 0; 0 1 0; 0 0 1]
  Transform String Midpoint : sm_lib/Frames and Transforms/Rigid Transform  TranslationMethod=StandardAxis  TranslationStandardOffset=L2/2  TranslationLengthUnit=m  TranslationStandardAxis=-Y  TranslationCartesianOffset=[0 0 0]  TranslationROffset=0  TranslationROffsetUnits=m  TranslationZOffset=0  TranslationZOffsetUnits=m  TranslationThetaOffset=0  TranslationThetaOffsetUnits=deg  RotationMethod=None  RotationAngleUnits=deg  RotationStandardAxis=+Z  RotationAngle=0  RotationArbitraryAxis=[0 0 1]  FollAlignAxisA=+X  BaseAlignAxisA=+Y  FollAlignAxisB=+Y  BaseAlignAxisB=+Z  RotationSequenceAxes=FollowerAxes  RotationSequence=XYX  RotationSequenceAngles=[0 0 0]  RotationSequenceAnglesUnits=deg  RotationMatrix=[1 0 0; 0 1 0; 0 0 1]
  B : PMIOPort  Side=Right
  F : PMIOPort  Port=2  Side=Left
  connections:
  Transform String Midpoint/RConn1 -- String/RConn1
  "Transform Bob "/RConn1 -- F/RConn1 -- Bob/RConn1
  B/RConn1 -- Transform String Midpoint/LConn1 -- "Transform Bob "/LConn1

== system Coupled_GP_fit/2 link pendulum/Pivot ==
  Base : sm_lib/Body Elements/Solid  InertiaType=CalculateFromGeometry  Mass=1  MassUnits=kg  CenterOfMass=[0 0 0]  CenterOfMassUnits=m  MomentsOfInertia=[1 1 1]*1e-3  MomentsOfInertiaUnits=kg*m^2  ProductsOfInertia=[0 0 0]  ProductsOfInertiaUnits=kg*m^2  BasedOnType=Density  Density=1000  DensityUnits=kg/(m^3)  DoExposeReferenceFrame=on  SerializedFrames=<Frames/>  GraphicType=FromGeometry  MarkerShape=Sphere  MarkerSize=10  MarkerSizeUnits=m  GraphicVisPropType=SimpleVisualProperties  GraphicDiffuseColor=[0.2 0.2 0.2]  GraphicSpecularColor=[0.5 0.5 0.5 1.0]  GraphicAmbientColor=[0.15 0.15 0.15 1.0]  GraphicEmissiveColor=[0.0 0.0 0.0 1.0]  GraphicShininess=75  GraphicOpacity=1.0  GeometryShape=Cylinder  RectangleSize=[1 1]  RectangleSizeUnits=m  BrickDimensions=[1 0.1 0.1]  BrickDimensionUnits=m  CylinderRadius=0.1  CylinderRadiusUnits=m  CylinderLength=0.1  CylinderLengthUnits=m  SphereRadius=0.1  SphereRadiusUnits=m  EllipsoidRadii=[1 1 1]  EllipsoidRadiiUnits=m  ExtrusionCrossSection=[1 1; -1 1; -1 -1; 1 -1]  ExtrusionCrossSectionUnits=m  ExtrusionLength=1  ExtrusionLengthUnits=m  PolygonNumSides=3  PolygonOuterRadius=1  PolygonOuterRadiusUnits=m  ExtGeomFileType=STL  ExtGeomFileUnits=m  RevolutionCrossSection=[1 1; 1 -1; 2 -1; 2 1]  RevolutionCrossSectionUnits=m  RevolutionExtent=Full  RevolutionAngle=180  RevolutionAngleUnits=deg
  Mechanism Configuration : sm_lib/Utilities/Mechanism Configuration  UniformGravity=Constant  GravityVector=[0 -g 0]  GravityUnits=m/s^2  LinearizationDelta=0.001
  Solver Configuration : nesl_utility/Solver Configuration  PhysicalDomain=network_engine_domain  SubClassName=solver  LeftPortType=input  RightPortType=generic  Tones=[]  Harmonics=[]  SimulateNoise=off  Profile=off  UseLocalSampling=off  EnableSwitchedLinearOptims=on  FrequencyDomain=off  UseCCode=off  RelTol=0.001  AbsTol=1e-06  MinStep=1e-09  ToWorkspace=off  RevertToSquareIcSolve=off  NumHomotopyIterations=100  PhasorMode=off  PhasorModeNumHarmonics=1  DoDC=off  ResidualTolerance=1e-9  UseLocalSolver=off  LocalSolverChoice=NE_BACKWARD_EULER_ADVANCER  LocalSolverSampleTime=.001  DoFixedCost=off  MaxNonlinIter=3  MaxModeIter=2  LinearAlgebra=Sparse  EquationFormulation=NE_TIME_EF  DelaysMemoryBudget=1024  AutomaticFiltering=on  FilteringTimeConstant=0.001  PartitionStorageMethod=AS_NEEDED  PartitionMemoryBudget=1024
  W : PMIOPort  Side=Left
  B : PMIOPort  Port=2  Side=Right
  connections:
  W/RConn1 -- B/RConn1 -- Base/RConn1 -- Solver Configuration/RConn1 -- Mechanism Configuration/RConn1

== system Coupled_GP_fit/Controller/PID 1 ==
  In1 : Inport
  Discrete-Time Integrator : DiscreteIntegrator  SampleTime=ts  ICPrevOutput=DiscIntNeverNeededParam  ICPrevScaledInput=DiscIntNeverNeededParam
  Discrete-Time Integrator1 : DiscreteIntegrator  IntegratorMethod=Integration: Trapezoidal  SampleTime=ts  UpperSaturationLimit=I_limit  LowerSaturationLimit=-I_limit  ICPrevOutput=DiscIntNeverNeededParam  ICPrevScaledInput=DiscIntNeverNeededParam
  Gain : Gain  Gain=1/PID(1).tau_p
  Sum : Sum  Inputs=|+-
  Sum1 : Sum  Inputs=+++
  kd : Gain  Gain=PID(1).kp*PID(1).tau_z
  ki : Gain  Gain=PID(1).kp/PID(1).tau_i
  kp : Gain  Gain=PID(1).kp*(1+PID(1).tau_z/PID(1).tau_i)
  Out1 : Outport
  wires:
  In1/1 -> Sum/1
  Gain/1 -> kd/1, Discrete-Time Integrator/1
  Sum1/1 -> Out1/1
  Discrete-Time Integrator/1 -> kp/1, ki/1, Sum/2
  Discrete-Time Integrator1/1 -> Sum1/3
  kp/1 -> Sum1/2
  ki/1 -> Discrete-Time Integrator1/1
  kd/1 -> Sum1/1
  Sum/1 -> Gain/1

== system Coupled_GP_fit/Controller/PID 2 ==
  In1 : Inport
  Discrete-Time Integrator : DiscreteIntegrator  SampleTime=ts  ICPrevOutput=DiscIntNeverNeededParam  ICPrevScaledInput=DiscIntNeverNeededParam
  Discrete-Time Integrator1 : DiscreteIntegrator  IntegratorMethod=Integration: Trapezoidal  SampleTime=ts  UpperSaturationLimit=I_limit  LowerSaturationLimit=-I_limit  ICPrevOutput=DiscIntNeverNeededParam  ICPrevScaledInput=DiscIntNeverNeededParam
  Gain : Gain  Gain=1/PID(2).tau_p
  Sum : Sum  Inputs=|+-
  Sum1 : Sum  Inputs=+++
  kd : Gain  Gain=PID(2).kp*PID(2).tau_z
  ki : Gain  Gain=PID(2).kp/PID(2).tau_i
  kp : Gain  Gain=PID(2).kp*(1+PID(2).tau_z/PID(2).tau_i)
  Out1 : Outport
  wires:
  In1/1 -> Sum/1
  Gain/1 -> kd/1, Discrete-Time Integrator/1
  Sum1/1 -> Out1/1
  Discrete-Time Integrator/1 -> kp/1, ki/1, Sum/2
  Discrete-Time Integrator1/1 -> Sum1/3
  kp/1 -> Sum1/2
  ki/1 -> Discrete-Time Integrator1/1
  kd/1 -> Sum1/1
  Sum/1 -> Gain/1

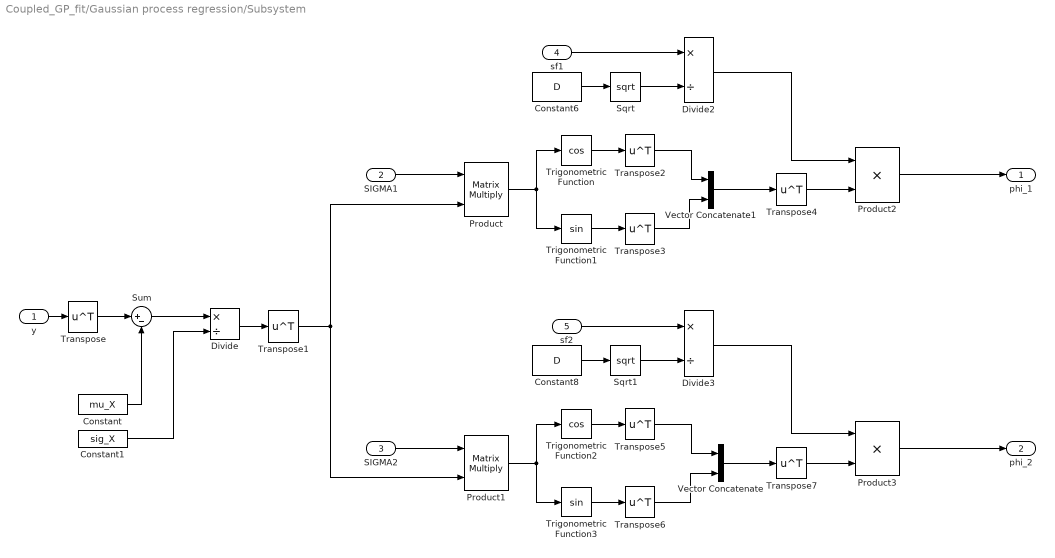
== system Coupled_GP_fit/Gaussian process regression/Subsystem ==
  y : Inport
  SIGMA1 : Inport  Port=2
  SIGMA2 : Inport  Port=3
  sf1 : Inport  Port=4
  sf2 : Inport  Port=5
  Constant : Constant  Value=mu_X  VectorParams1D=off  SampleTime=-1
  Constant1 : Constant  Value=sig_X  VectorParams1D=off  SampleTime=-1
  Constant6 : Constant  Value=D  SampleTime=-1
  Constant8 : Constant  Value=D  SampleTime=-1
  Divide : Product  Inputs=*/
  Divide2 : Product  Inputs=*/
  Divide3 : Product  Inputs=*/
  Product : Product  Multiplication=Matrix(*)
  Product1 : Product  Multiplication=Matrix(*)
  Product2 : Product
  Product3 : Product
  Sqrt : Sqrt  SaturateOnIntegerOverflow=on
  Sqrt1 : Sqrt  SaturateOnIntegerOverflow=on
  Sum : Sum  Inputs=|+-
  Transpose{,1..7} (8 alike) : Math  Operator=transpose  SaturateOnIntegerOverflow=on
  Trigonometric Function : Trigonometry  Operator=cos
  Trigonometric Function1 : Trigonometry
  Trigonometric Function2 : Trigonometry  Operator=cos
  Trigonometric Function3 : Trigonometry
  Vector Concatenate : Concatenate
  Vector Concatenate1 : Concatenate
  phi_1 : Outport
  phi_2 : Outport  Port=2
  wires:
  sf2/1 -> Divide3/1
  Transpose5/1 -> Vector Concatenate/1
  Transpose1/1 -> Product/2, Product1/2
  Divide3/1 -> Product3/1
  Divide/1 -> Transpose1/1
  Product1/1 -> Trigonometric Function3/1, Trigonometric Function2/1
  y/1 -> Transpose/1
  Product/1 -> Trigonometric Function1/1, Trigonometric Function/1
  Product2/1 -> phi_1/1
  sf1/1 -> Divide2/1
  Divide2/1 -> Product2/1
  Sum/1 -> Divide/1
  Constant1/1 -> Divide/2
  Constant/1 -> Sum/2
  Constant8/1 -> Sqrt1/1
  Sqrt1/1 -> Divide3/2
  Transpose7/1 -> Product3/2
  Transpose6/1 -> Vector Concatenate/2
  Transpose2/1 -> Vector Concatenate1/1
  Transpose4/1 -> Product2/2
  Constant6/1 -> Sqrt/1
  Product3/1 -> phi_2/1
  Vector Concatenate/1 -> Transpose7/1
  Trigonometric Function1/1 -> Transpose3/1
  Trigonometric Function2/1 -> Transpose5/1
  Trigonometric Function3/1 -> Transpose6/1
  Trigonometric Function/1 -> Transpose2/1
  Vector Concatenate1/1 -> Transpose4/1
  Transpose3/1 -> Vector Concatenate1/2
  Sqrt/1 -> Divide2/2
  SIGMA2/1 -> Product1/1
  SIGMA1/1 -> Product/1
  Transpose/1 -> Sum/1

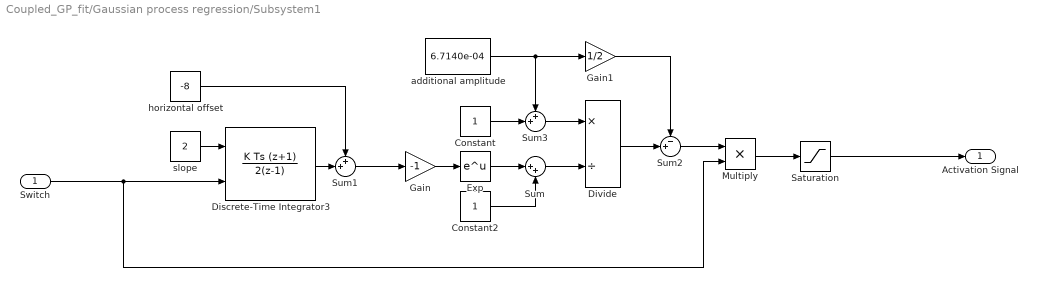
== system Coupled_GP_fit/Gaussian process regression/Subsystem1 ==
  Switch : Inport
  Constant : Constant
  Constant2 : Constant
  Discrete-Time Integrator3 : DiscreteIntegrator  IntegratorMethod=Integration: Trapezoidal  ExternalReset=rising  SampleTime=-1  UpperSaturationLimit=1  LowerSaturationLimit=0  ICPrevOutput=DiscIntNeverNeededParam  ICPrevScaledInput=DiscIntNeverNeededParam
  Divide : Product  Inputs=*/
  Exp : Math  SaturateOnIntegerOverflow=on
  Gain : Gain  Gain=-1
  Gain1 : Gain  Gain=1/2
  Multiply : Product
  Saturation : Saturate  UpperLimit=1  LowerLimit=0
  Sum : Sum  Inputs=|++
  Sum1 : Sum  Inputs=++|
  Sum2 : Sum  Inputs=-+|
  Sum3 : Sum  Inputs=++|
  additional amplitude : Constant  Value=6.7140e-04
  horizontal offset : Constant  Value=-8
  slope : Constant  Value=2
  Activation Signal : Outport
  wires:
  Constant/1 -> Sum3/2
  Exp/1 -> Sum/1
  additional amplitude/1 -> Sum3/1, Gain1/1
  Sum1/1 -> Gain/1
  Gain1/1 -> Sum2/1
  Divide/1 -> Sum2/2
  Sum/1 -> Divide/2
  Gain/1 -> Exp/1
  slope/1 -> Discrete-Time Integrator3/1
  Discrete-Time Integrator3/1 -> Sum1/2
  Constant2/1 -> Sum/2
  Sum2/1 -> Multiply/1
  Sum3/1 -> Divide/1
  horizontal offset/1 -> Sum1/1
  Saturation/1 -> Activation Signal/1
  Multiply/1 -> Saturation/1
  Switch/1 -> Multiply/2, Discrete-Time Integrator3/2

== system Coupled_GP_fit/Setpoint Generator/TDfhan ==
  V : Inport
  Constant : Constant  Value=r
  Constant1 : Constant  Value=h
  Discrete-Time Integrator : DiscreteIntegrator  gainval=1  SampleTime=ts  ICPrevOutput=DiscIntNeverNeededParam  ICPrevScaledInput=DiscIntNeverNeededParam
  Discrete-Time Integrator1 : DiscreteIntegrator  gainval=1  SampleTime=ts  ICPrevOutput=DiscIntNeverNeededParam  ICPrevScaledInput=DiscIntNeverNeededParam
  MATLAB Function2 : MATLAB Function  TreatAsAtomicUnit=on
  Scope : Scope  NumInputPorts=3
  Sum : Sum  Inputs=+-|
  V1 : Outport
  V2 : Outport  Port=2
  V3 : Outport  Port=3
  wires:
  Discrete-Time Integrator/1 -> Discrete-Time Integrator1/1, MATLAB Function2/2(v2), Scope/2, V2/1  "V2"
  Discrete-Time Integrator1/1 -> Scope/1, V1/1, Sum/1  "V1"
  MATLAB Function2/1(output) -> Discrete-Time Integrator/1, V3/1, Scope/3  "fv"
  Sum/1 -> MATLAB Function2/1(v1)
  V/1 -> Sum/2
  Constant/1 -> MATLAB Function2/3(r0)
  Constant1/1 -> MATLAB Function2/4(h0)
